simulink model "gm_uz_mpc_delay_comp"  (R2021a)
settings: Solver=FixedStepDiscrete  StartTime=0.0  StopTime=1/f  RelTol=1e-3
undefined symbols (not defined in the file or in its folder): A, f, Ld_over_LB, Lq_over_LB, omega_m, omegaB, psi_pm_over_psiB, Rs_over_ZB, t_ADC, Ts_times_ZB_over_Ld, Ts_times_ZB_over_Lq, Ts_times_ZB_over_Lx, Ts_times_ZB_over_Ly, v_dc, VB
libraries: hdlmdlgenlib x44, fl_lib x7, nesl_utility x7, simulink x4, ee_lib x2, hdlsllib x1
settings Model: Creator=micha  LastModifiedBy=micha
settings SolverCC: AlgebraicLoopSolver=TrustRegion
settings DataIOCC: LimitDataPoints=on  SaveOutput=off  SaveTime=off
settings OptimizationCC: BlockReduction=off  ConditionallyExecuteInputs=off  DefaultParameterBehavior=Inlined  LifeSpan=inf
settings DebuggingCC: AlgebraicLoopMsg=error  InheritedTsInSrcMsg=none  SingleTaskRateTransMsg=error  AllowSymbolicDim=off  StrictBusMsg=ErrorOnBusTreatedAsVector  SFUnexpectedBacktrackingDiag=warning  SFNoUnconditionalDefaultTransitionDiag=warning  SFExecutionAtInitializationDiag=none  SFMachineParentedDataDiag=warning  ArithmeticOperatorsInVariantConditions=warning
settings HardwareCC: ProdBitPerPointer=32  ProdBitPerSizeT=32  ProdBitPerPtrDiffT=32  ProdLargestAtomicFloat=None  ProdIntDivRoundTo=Undefined  ProdEndianess=Unspecified  ProdWordSize=32  ProdHWDeviceType=ASIC/FPGA->ASIC/FPGA  ProdEqTarget=off
settings SFSimCC: SimUseLocalCustomCode=off  CustomCodeUndefinedFunction=UseInterfaceOnly
settings RTWCC: RTWUseLocalCustomCode=off
settings CodeAppCC: StateflowObjectComments=on
settings GRTTargetCC: TargetLangStandard=C89/C90 (ANSI)
settings ConfigComp: CovScope=ReferencedModels  CovMetricSettings=dw  CovSaveCumulativeToWorkspaceVar=on  CovSaveSingleToWorkspaceVar=on  CovExternalEMLEnable=off  CovSFcnEnable=off

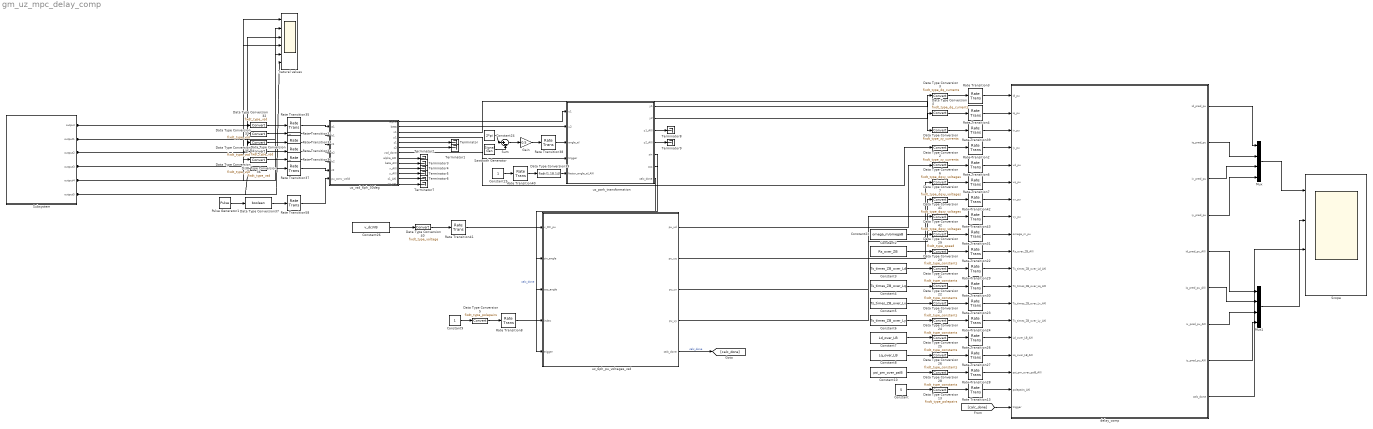
== system gm_uz_mpc_delay_comp ==
  Constant : Constant  Value=5
  Constant10 : Constant  Value=psi_pm_over_psiB
  Constant2 : Constant  Value=Rs_over_ZB
  Constant23 : Constant  Value=omega_m/omegaB
  Constant24 : Constant  Value=2*pi
  Constant25 : Constant
  Constant26 : Constant  Value=v_dc/VB
  Constant3 : Constant  Value=Ts_times_ZB_over_Ld
  Constant4 : Constant  Value=Ts_times_ZB_over_Lq
  Constant5 : Constant  Value=Ts_times_ZB_over_Lx
  Constant6 : Constant  Value=Ts_times_ZB_over_Ly
  Constant7 : Constant  Value=Ld_over_LB
  Constant8 : Constant  Value=Lq_over_LB
  Constant9 : Constant
  Data Type Conversion : DataTypeConversion  OutDataTypeStr=fixdt_type_xy_currents
  Data Type Conversion13 : DataTypeConversion  OutDataTypeStr=fixdt_type_polepairs
  Data Type Conversion2 : DataTypeConversion  OutDataTypeStr=fixdt_type_xy_currents
  Data Type Conversion{20..26,28} (8 alike) : DataTypeConversion  OutDataTypeStr=fixdt_type_constants
  Data Type Conversion29 : DataTypeConversion  OutDataTypeStr=fixdt_type_speed
  Data Type Conversion3 : DataTypeConversion  OutDataTypeStr=fixdt_type_dq_currents
  Data Type Conversion{32..36,38} (6 alike) : DataTypeConversion  OutDataTypeStr=fixdt_type_vsd
  Data Type Conversion37 : DataTypeConversion  OutDataTypeStr=boolean
  Data Type Conversion39 : DataTypeConversion  OutDataTypeStr=fixdt(1,18,14)
  Data Type Conversion4 : DataTypeConversion  OutDataTypeStr=fixdt_type_dq_currents
  Data Type Conversion40 : DataTypeConversion  OutDataTypeStr=fixdt_type_voltage
  Data Type Conversion{6..7,41..42} (4 alike) : DataTypeConversion  OutDataTypeStr=fixdt_type_dqxy_voltages
  Data Type Conversion5 : DataTypeConversion  OutDataTypeStr=fixdt_type_polepairs
  Gain : Gain  Gain=0.5
  Mux : Mux
  Mux1 : Mux
  Pulse Generator1 : DiscretePulseGenerator  PulseType=Time based  Period=t_ADC  PulseWidth=5
  Rate Transition{2..4,6..7,13,22..24,26..43,58} (28 alike) : RateTransition  OutPortSampleTime=t_clock
  Rate Transition8 : RateTransition  InitialCondition=1  OutPortSampleTime=t_clock
  Sawtooth Generator : SignalGenerator  WaveForm=sawtooth  Amplitude=2*pi  Frequency=2*pi*f  Units=rad/sec
  Scope : Scope  NumInputPorts=4
  Subsystem : Subsystem
  Sum : Sum  Inputs=|+-
  Terminator{,1..9} (10 alike) : Terminator
  delay_comp : Subsystem  TreatAsAtomicUnit=on
  natural values : Scope  NumInputPorts=6
  uz_6ph_pu_voltages_vsd : Subsystem
  uz_park_transformation : Subsystem  TreatAsAtomicUnit=on
  uz_vsd_6ph_30deg : Subsystem  TreatAsAtomicUnit=on
  wires:
  Data Type Conversion5/1 -> Rate Transition8/1
  Constant9/1 -> Data Type Conversion5/1
  Rate Transition8/1 -> uz_6ph_pu_voltages_vsd/4(index)
  delay_comp/9(calc_done) -> Scope/3
  Mux1/1 -> Scope/2
  delay_comp/5(id_pred_pu_AXI) -> Mux1/1
  delay_comp/7(ix_pred_pu_AXI) -> Mux1/3
  delay_comp/8(iy_pred_pu_AXI) -> Mux1/4
  delay_comp/6(iq_pred_pu_AXI) -> Mux1/2
  Mux/1 -> Scope/1
  delay_comp/4(iy_pred_pu) -> Mux/4
  delay_comp/3(ix_pred_pu) -> Mux/3
  delay_comp/2(iq_pred_pu) -> Mux/2
  delay_comp/1(id_pred_pu) -> Mux/1
  Rate Transition13/1 -> delay_comp/18(polepairs_AXI)
  Data Type Conversion13/1 -> Rate Transition13/1
  Constant/1 -> Data Type Conversion13/1
  Rate Transition28/1 -> delay_comp/17(psi_pm_over_psiB_AXI)
  Data Type Conversion28/1 -> Rate Transition28/1
  Constant10/1 -> Data Type Conversion28/1
  [calc_done] -> delay_comp/19(trigger)
  Rate Transition34/1 -> uz_vsd_6ph_30deg/4(a2)
  Data Type Conversion37/1 -> Rate Transition58/1
  Data Type Conversion36/1 -> Rate Transition36/1
  Constant26/1 -> Data Type Conversion40/1
  Data Type Conversion35/1 -> Rate Transition34/1
  uz_vsd_6ph_30deg/5(z1) -> Terminator/1
  uz_vsd_6ph_30deg/3(x1) -> Data Type Conversion/1
  Data Type Conversion32/1 -> Rate Transition35/1
  Data Type Conversion33/1 -> Rate Transition32/1
  Subsystem/6(output5) -> Data Type Conversion38/1, natural values/6
  Rate Transition32/1 -> uz_vsd_6ph_30deg/2(b1)
  Subsystem/3(output2) -> natural values/3, Data Type Conversion34/1
  Data Type Conversion34/1 -> Rate Transition33/1
  Rate Transition40/1 -> Data Type Conversion39/1
  Constant25/1 -> Rate Transition40/1
  Sawtooth Generator/1 -> Sum/2
  Rate Transition58/1 -> uz_vsd_6ph_30deg/7(pu_conv_valid)
  Sum/1 -> Gain/1
  Rate Transition36/1 -> uz_vsd_6ph_30deg/5(b2)
  Gain/1 -> Rate Transition38/1
  Subsystem/4(output3) -> natural values/4, Data Type Conversion35/1
  Data Type Conversion38/1 -> Rate Transition37/1
  Rate Transition38/1 -> uz_park_transformation/3(angle_el)
  uz_6ph_pu_voltages_vsd/1(pu_ud) -> Data Type Conversion6/1
  uz_6ph_pu_voltages_vsd/3(pu_ux) -> Data Type Conversion41/1
  Rate Transition33/1 -> uz_vsd_6ph_30deg/3(c1)
  uz_6ph_pu_voltages_vsd/5(calc_done) -> [calc_done]  "calc_done"
  Subsystem/5(output4) -> natural values/5, Data Type Conversion36/1
  uz_vsd_6ph_30deg/9(beta_AXI) -> Terminator3/1
  uz_park_transformation/1(y1) -> Data Type Conversion3/1
  uz_vsd_6ph_30deg/6(z2) -> Terminator1/1
  uz_vsd_6ph_30deg/10(x_AXI) -> Terminator4/1
  Rate Transition37/1 -> uz_vsd_6ph_30deg/6(c2)
  uz_vsd_6ph_30deg/4(y1) -> Data Type Conversion2/1
  Rate Transition41/1 -> uz_6ph_pu_voltages_vsd/1(v_DC_pu)
  uz_vsd_6ph_30deg/1(alpha) -> uz_park_transformation/1(u1)
  uz_park_transformation/6(cos) -> uz_6ph_pu_voltages_vsd/3(cos_angle)
  uz_park_transformation/7(calc_done) -> uz_6ph_pu_voltages_vsd/5(trigger)  "calc_done"
  Data Type Conversion39/1 -> uz_park_transformation/5(factor_angle_el_AXI)
  uz_6ph_pu_voltages_vsd/4(pu_uy) -> Data Type Conversion42/1
  uz_vsd_6ph_30deg/7(vsd_done) -> uz_park_transformation/4(trigger)
  Subsystem/2(output1) -> Data Type Conversion33/1, natural values/2
  Pulse Generator1/1 -> Data Type Conversion37/1
  uz_park_transformation/5(sin) -> uz_6ph_pu_voltages_vsd/2(sin_angle)
  Rate Transition35/1 -> uz_vsd_6ph_30deg/1(a1)
  uz_6ph_pu_voltages_vsd/2(pu_uq) -> Data Type Conversion7/1
  uz_vsd_6ph_30deg/2(beta) -> uz_park_transformation/2(u2)
  Constant24/1 -> Sum/1
  Data Type Conversion40/1 -> Rate Transition41/1
  Subsystem/1(output) -> Data Type Conversion32/1, natural values/1
  uz_park_transformation/2(y2) -> Data Type Conversion4/1
  uz_vsd_6ph_30deg/11(y_AXI) -> Terminator5/1
  uz_park_transformation/3(y1_AXI) -> Terminator8/1
  uz_vsd_6ph_30deg/13(z2_AXI) -> Terminator7/1
  uz_vsd_6ph_30deg/8(alpha_AXI) -> Terminator2/1
  uz_park_transformation/4(y2_AXI) -> Terminator9/1
  uz_vsd_6ph_30deg/12(z1_AXI) -> Terminator6/1
  Rate Transition43/1 -> delay_comp/8(vy_pu)
  Rate Transition7/1 -> delay_comp/6(vq_pu)
  Rate Transition6/1 -> delay_comp/5(vd_pu)
  Data Type Conversion42/1 -> Rate Transition43/1
  Data Type Conversion7/1 -> Rate Transition7/1
  Data Type Conversion41/1 -> Rate Transition42/1
  Rate Transition42/1 -> delay_comp/7(vx_pu)
  Data Type Conversion6/1 -> Rate Transition6/1
  Rate Transition39/1 -> delay_comp/3(ix_pu)
  Rate Transition4/1 -> delay_comp/2(iq_pu)
  Data Type Conversion2/1 -> Rate Transition2/1
  Data Type Conversion/1 -> Rate Transition39/1
  Data Type Conversion4/1 -> Rate Transition4/1
  Rate Transition3/1 -> delay_comp/1(id_pu)
  Data Type Conversion3/1 -> Rate Transition3/1
  Rate Transition2/1 -> delay_comp/4(iy_pu)
  Rate Transition31/1 -> delay_comp/9(omega_m_pu)
  Constant23/1 -> Data Type Conversion29/1
  Data Type Conversion29/1 -> Rate Transition31/1
  Constant7/1 -> Data Type Conversion25/1
  Constant4/1 -> Data Type Conversion22/1
  Constant5/1 -> Data Type Conversion23/1
  Rate Transition23/1 -> delay_comp/13(Ts_times_ZB_over_Lx_AXI)
  Data Type Conversion20/1 -> Rate Transition22/1
  Rate Transition24/1 -> delay_comp/14(Ts_times_ZB_over_Ly_AXI)
  Rate Transition26/1 -> delay_comp/15(Ld_over_LB_AXI)
  Data Type Conversion23/1 -> Rate Transition23/1
  Data Type Conversion22/1 -> Rate Transition30/1
  Data Type Conversion25/1 -> Rate Transition26/1
  Constant2/1 -> Data Type Conversion20/1
  Constant3/1 -> Data Type Conversion21/1
  Rate Transition27/1 -> delay_comp/16(Lq_over_LB_AXI)
  Rate Transition30/1 -> delay_comp/12(Ts_times_ZB_over_Lq_AXI)
  Constant6/1 -> Data Type Conversion24/1
  Data Type Conversion26/1 -> Rate Transition27/1
  Rate Transition29/1 -> delay_comp/11(Ts_times_ZB_over_Ld_AXI)
  Data Type Conversion21/1 -> Rate Transition29/1
  Rate Transition22/1 -> delay_comp/10(Rs_over_ZB_AXI)
  Constant8/1 -> Data Type Conversion26/1
  Data Type Conversion24/1 -> Rate Transition24/1

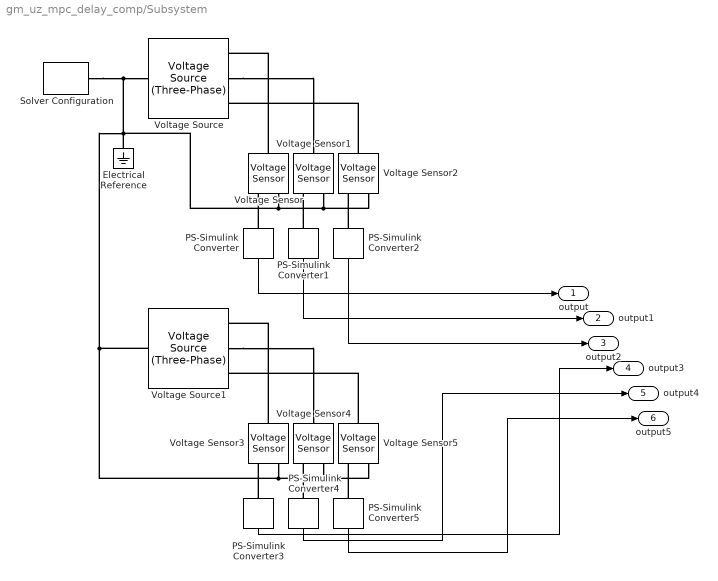
== system gm_uz_mpc_delay_comp/Subsystem ==
  Electrical Reference : fl_lib/Electrical/Electrical Elements/Electrical Reference
  PS-Simulink Converter{,1..5} (6 alike) : nesl_utility/PS-Simulink Converter  PhysicalDomain=network_engine_domain  SubClassName=ps_output  LeftPortType=input  RightPortType=output  PseudoPeriodic=off  Frequencies=[]  Unit=1  AffineConversion=off
  Solver Configuration : nesl_utility/Solver Configuration  PhysicalDomain=network_engine_domain  SubClassName=solver  LeftPortType=input  RightPortType=generic  Tones=[]  Harmonics=[]  SimulateNoise=off  Profile=off  UseLocalSampling=off  EnableSwitchedLinearOptims=on  FrequencyDomain=off  UseCCode=off  RelTol=0.001  AbsTol=1e-06  MinStep=1e-09  ToWorkspace=off  RevertToSquareIcSolve=off  NumHomotopyIterations=100  PhasorMode=off  PhasorModeNumHarmonics=1  DoDC=off  ResidualTolerance=1e-09  UseLocalSolver=on  LocalSolverChoice=NE_BACKWARD_EULER_ADVANCER  LocalSolverSampleTime=1e-6  DoFixedCost=on  MaxNonlinIter=3  MaxModeIter=2  ComputeImpulses=off  ImpulseIterations=2  LinearAlgebra=Sparse  EquationFormulation=NE_TIME_EF  DelaysMemoryBudget=1024  AutomaticFiltering=on  FilteringTimeConstant=0.001  PartitionStorageMethod=AS_NEEDED  PartitionMemoryBudget=1024  PartitionMethod=FAST
  Voltage Sensor{,1..5} (6 alike) : fl_lib/Electrical/Electrical Sensors/Voltage Sensor
  Voltage Source : ee_lib/Sources/Voltage Source (Three-Phase)  vline_rms=A*sqrt(3)/sqrt(2) V  shift=0 deg  freq=f Hz  impedance_option=1  SShortCircuit=1e6 V*A  XR=15  R=0.01 Ohm  L=3.97e-4 H  G_parasitic=0 1/Ohm  harmonic_option=1  harmonic_orders=Harmonic_Orders  harmonic_ratios=Harmonic_Amplitudes  I_specify=off  I_priority=None  I=[ 0 0 0 ] A  I_nominal_specify=off  I_nominal_unit=A  I_nominal_value=1
      settings: SourceProductBaseCode=PS  InternalSimscapePortConfiguration="{\"Bottom\":[],\"Left\":[{\"id\":\"n\",\"label\":\"n\",\"type\":\"foundation.electrical.electrical\"}],\"Right\":[{\"id\":\"a\",\"label\":\"a\",\"type\":\"foundation.electrical.electrical\"},{\"id\":\"b\",\"label\":\"b\",\"type\":\"foundation.electrical.electrical\"},{\"id\":\"c\",\"label\":\"c\",\"type\":\"foundation.electrical.electrical\"}],\"Top\":[]}"
  Voltage Source1 : ee_lib/Sources/Voltage Source (Three-Phase)  vline_rms=A*sqrt(3)/sqrt(2) V  shift=-30 deg  freq=f Hz  impedance_option=1  SShortCircuit=1e6 V*A  XR=15  R=0.01 Ohm  L=3.97e-4 H  G_parasitic=0 1/Ohm  harmonic_option=1  harmonic_orders=Harmonic_Orders  harmonic_ratios=Harmonic_Amplitudes  I_specify=off  I_priority=None  I=[ 0 0 0 ] A  I_nominal_specify=off  I_nominal_unit=A  I_nominal_value=1
      settings: SourceProductBaseCode=PS  InternalSimscapePortConfiguration="{\"Bottom\":[],\"Left\":[{\"id\":\"n\",\"label\":\"n\",\"type\":\"foundation.electrical.electrical\"}],\"Right\":[{\"id\":\"a\",\"label\":\"a\",\"type\":\"foundation.electrical.electrical\"},{\"id\":\"b\",\"label\":\"b\",\"type\":\"foundation.electrical.electrical\"},{\"id\":\"c\",\"label\":\"c\",\"type\":\"foundation.electrical.electrical\"}],\"Top\":[]}"
  output : Outport
  output1 : Outport  Port=2
  output2 : Outport  Port=3
  output3 : Outport  Port=4
  output4 : Outport  Port=5
  output5 : Outport  Port=6
  wires:
  PS-Simulink Converter2/1 -> output2/1
  PS-Simulink Converter5/1 -> output5/1
  PS-Simulink Converter1/1 -> output1/1
  PS-Simulink Converter4/1 -> output4/1
  PS-Simulink Converter3/1 -> output3/1
  PS-Simulink Converter/1 -> output/1
  connections:
  Voltage Source/RConn2 -- Voltage Sensor1/LConn1
  Voltage Sensor/LConn1 -- Voltage Source/RConn1
  PS-Simulink Converter3/LConn1 -- Voltage Sensor3/RConn1
  PS-Simulink Converter2/LConn1 -- Voltage Sensor2/RConn1
  Voltage Sensor2/LConn1 -- Voltage Source/RConn3
  PS-Simulink Converter4/LConn1 -- Voltage Sensor4/RConn1
  Voltage Sensor5/LConn1 -- Voltage Source1/RConn3
  Voltage Source1/RConn2 -- Voltage Sensor4/LConn1
  PS-Simulink Converter/LConn1 -- Voltage Sensor/RConn1
  Voltage Sensor3/LConn1 -- Voltage Source1/RConn1
  PS-Simulink Converter1/LConn1 -- Voltage Sensor1/RConn1
  PS-Simulink Converter5/LConn1 -- Voltage Sensor5/RConn1
  Voltage Sensor4/RConn2 -- Voltage Sensor3/RConn2 -- Voltage Source1/LConn1 -- Electrical Reference/LConn1 -- Voltage Sensor/RConn2 -- Voltage Sensor1/RConn2 -- Voltage Sensor2/RConn2 -- Voltage Source/LConn1 -- Solver Configuration/RConn1 -- Voltage Sensor5/RConn2

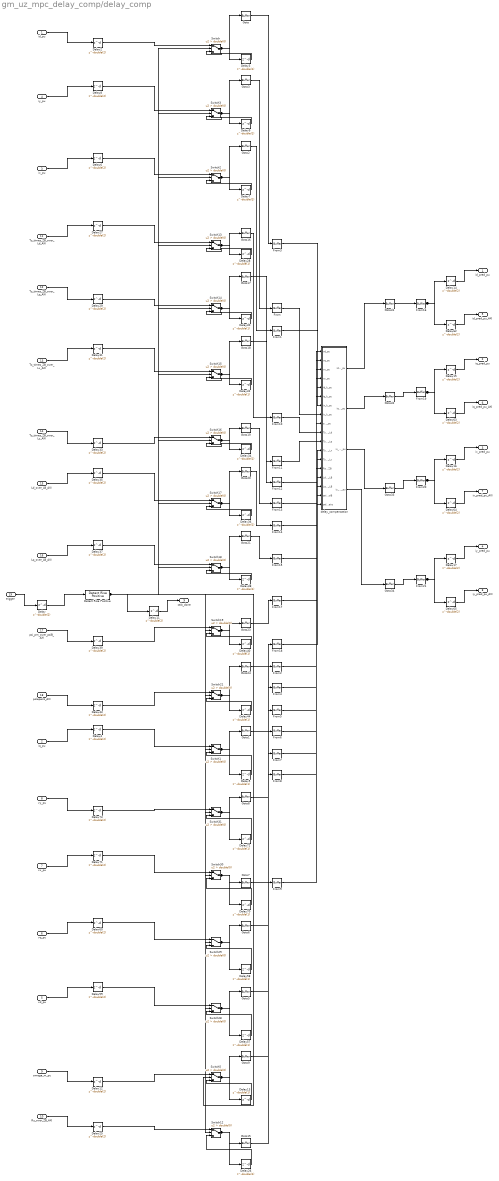
== system gm_uz_mpc_delay_comp/delay_comp ==
  id_pu : Inport  OutDataTypeStr=fixdt(1, 27, 16)  PortDimensions=1  SampleTime=1e-08
  iq_pu : Inport  Port=2  OutDataTypeStr=fixdt(1, 27, 16)  PortDimensions=1  SampleTime=1e-08
  ix_pu : Inport  Port=3  OutDataTypeStr=fixdt(1, 18, 11)  PortDimensions=1  SampleTime=1e-08
  iy_pu : Inport  Port=4  OutDataTypeStr=fixdt(1, 18, 11)  PortDimensions=1  SampleTime=1e-08
  vd_pu : Inport  Port=5  OutDataTypeStr=fixdt(1, 27, 24)  PortDimensions=1  SampleTime=1e-08
  vq_pu : Inport  Port=6  OutDataTypeStr=fixdt(1, 27, 24)  PortDimensions=1  SampleTime=1e-08
  vx_pu : Inport  Port=7  OutDataTypeStr=fixdt(1, 27, 24)  PortDimensions=1  SampleTime=1e-08
  vy_pu : Inport  Port=8  OutDataTypeStr=fixdt(1, 27, 24)  PortDimensions=1  SampleTime=1e-08
  omega_m_pu : Inport  Port=9  OutDataTypeStr=fixdt(1, 18, 15)  PortDimensions=1  SampleTime=1e-08
  Rs_over_ZB_AXI : Inport  Port=10  OutDataTypeStr=fixdt(1, 18, 15)  PortDimensions=1  SampleTime=1e-08
  Ts_times_ZB_over_Ld_AXI : Inport  Port=11  OutDataTypeStr=fixdt(1, 18, 15)  PortDimensions=1  SampleTime=1e-08
  Ts_times_ZB_over_Lq_AXI : Inport  Port=12  OutDataTypeStr=fixdt(1, 18, 15)  PortDimensions=1  SampleTime=1e-08
  Ts_times_ZB_over_Lx_AXI : Inport  Port=13  OutDataTypeStr=fixdt(1, 18, 15)  PortDimensions=1  SampleTime=1e-08
  Ts_times_ZB_over_Ly_AXI : Inport  Port=14  OutDataTypeStr=fixdt(1, 18, 15)  PortDimensions=1  SampleTime=1e-08
  Ld_over_LB_AXI : Inport  Port=15  OutDataTypeStr=fixdt(1, 18, 15)  PortDimensions=1  SampleTime=1e-08
  Lq_over_LB_AXI : Inport  Port=16  OutDataTypeStr=fixdt(1, 18, 15)  PortDimensions=1  SampleTime=1e-08
  psi_pm_over_psiB_AXI : Inport  Port=17  OutDataTypeStr=fixdt(1, 18, 15)  PortDimensions=1  SampleTime=1e-08
  polepairs_AXI : Inport  Port=18  OutDataTypeStr=uint32  PortDimensions=1  SampleTime=1e-08
  trigger : Inport  Port=19  OutDataTypeStr=boolean  PortDimensions=1  SampleTime=1e-08
  Delay{,2,4,6,8,11..12,14..17,25,27,29,31,33,35,37,39,43,59..60,62..65,71,73} (28 alike) : Delay  DelayLength=double(2)  InitialCondition=0  SampleTime=1e-08
  Delay{3,5,7,9,13,26,28,30,32,34,36,38,40,44,57..58,70,72} (18 alike) : Delay  DelayLength=double(1)  InitialCondition=0  SampleTime=1e-08
  Detect Rise Positive : simulink/Logic and Bit Operations/Detect Rise Positive  vinit=0  OutDataTypeStr=boolean
  From{,1..21} (22 alike) : hdlmdlgenlib/Buffer
      settings: SourceProductBaseCode=SL
  Goto{,1..3,5..9,15..21,23..24,31..34} (22 alike) : hdlmdlgenlib/Buffer
      settings: SourceProductBaseCode=SL
  Switch : Switch  Criteria=u2 > Threshold  Threshold=double(0)  OutDataTypeStr=fixdt(1, 27, 16)  SampleTime=1e-08
  Switch1 : Switch  Criteria=u2 > Threshold  Threshold=double(0)  OutDataTypeStr=fixdt(1, 27, 16)  SampleTime=1e-08
  Switch{5,12..19} (9 alike) : Switch  Criteria=u2 > Threshold  Threshold=double(0)  OutDataTypeStr=fixdt(1, 18, 15)  SampleTime=1e-08
  Switch2 : Switch  Criteria=u2 > Threshold  Threshold=double(0)  OutDataTypeStr=fixdt(1, 18, 11)  SampleTime=1e-08
  Switch21 : Switch  Criteria=u2 > Threshold  Threshold=double(0)  OutDataTypeStr=uint32  SampleTime=1e-08
  Switch{28..31} (4 alike) : Switch  Criteria=u2 > Threshold  Threshold=double(0)  OutDataTypeStr=fixdt(1, 27, 24)  SampleTime=1e-08
  Switch3 : Switch  Criteria=u2 > Threshold  Threshold=double(0)  OutDataTypeStr=fixdt(1, 18, 11)  SampleTime=1e-08
  delay_compensation : Subsystem
  id_pred_pu : Outport  SampleTime=1e-08
  iq_pred_pu : Outport  Port=2  SampleTime=1e-08
  ix_pred_pu : Outport  Port=3  SampleTime=1e-08
  iy_pred_pu : Outport  Port=4  SampleTime=1e-08
  id_pred_pu_AXI : Outport  Port=5  SampleTime=1e-08
  iq_pred_pu_AXI : Outport  Port=6  SampleTime=1e-08
  ix_pred_pu_AXI : Outport  Port=7  SampleTime=1e-08
  iy_pred_pu_AXI : Outport  Port=8  SampleTime=1e-08
  calc_done : Outport  Port=9  SampleTime=1e-08
  wires:
  id_pu/1 -> Delay2/1
  iq_pu/1 -> Delay4/1
  ix_pu/1 -> Delay6/1
  iy_pu/1 -> Delay8/1
  vd_pu/1 -> Delay59/1
  vq_pu/1 -> Delay60/1
  vx_pu/1 -> Delay71/1
  vy_pu/1 -> Delay73/1
  omega_m_pu/1 -> Delay12/1
  Rs_over_ZB_AXI/1 -> Delay25/1
  Ts_times_ZB_over_Ld_AXI/1 -> Delay27/1
  Ts_times_ZB_over_Lq_AXI/1 -> Delay29/1
  Ts_times_ZB_over_Lx_AXI/1 -> Delay31/1
  Ts_times_ZB_over_Ly_AXI/1 -> Delay33/1
  Ld_over_LB_AXI/1 -> Delay35/1
  Lq_over_LB_AXI/1 -> Delay37/1
  psi_pm_over_psiB_AXI/1 -> Delay39/1
  polepairs_AXI/1 -> Delay43/1
  trigger/1 -> Delay/1
  Delay/1 -> Detect Rise Positive/1
  Delay11/1 -> calc_done/1
  Delay12/1 -> Switch5/1
  Delay13/1 -> Switch5/3
  Delay14/1 -> id_pred_pu/1
  Delay15/1 -> iq_pred_pu/1
  Delay16/1 -> ix_pred_pu/1
  Delay17/1 -> iy_pred_pu/1
  Delay2/1 -> Switch/1
  Delay25/1 -> Switch12/1
  Delay26/1 -> Switch12/3
  Delay27/1 -> Switch13/1
  Delay28/1 -> Switch13/3
  Delay29/1 -> Switch14/1
  Delay3/1 -> Switch/3
  Delay30/1 -> Switch14/3
  Delay31/1 -> Switch15/1
  Delay32/1 -> Switch15/3
  Delay33/1 -> Switch16/1
  Delay34/1 -> Switch16/3
  Delay35/1 -> Switch17/1
  Delay36/1 -> Switch17/3
  Delay37/1 -> Switch18/1
  Delay38/1 -> Switch18/3
  Delay39/1 -> Switch19/1
  Delay4/1 -> Switch1/1
  Delay40/1 -> Switch19/3
  Delay43/1 -> Switch21/1
  Delay44/1 -> Switch21/3
  Delay5/1 -> Switch1/3
  Delay57/1 -> Switch28/3
  Delay58/1 -> Switch29/3
  Delay59/1 -> Switch28/1
  Delay6/1 -> Switch2/1
  Delay60/1 -> Switch29/1
  Delay62/1 -> id_pred_pu_AXI/1
  Delay63/1 -> iq_pred_pu_AXI/1
  Delay64/1 -> ix_pred_pu_AXI/1
  Delay65/1 -> iy_pred_pu_AXI/1
  Delay7/1 -> Switch2/3
  Delay70/1 -> Switch30/3
  Delay71/1 -> Switch30/1
  Delay72/1 -> Switch31/3
  Delay73/1 -> Switch31/1
  Delay8/1 -> Switch3/1
  Delay9/1 -> Switch3/3
  Detect Rise Positive/1 -> Switch5/2, Switch31/2, Switch30/2, Switch3/2, Switch29/2, Switch28/2, Switch21/2, Switch2/2, Switch19/2, Switch18/2, Switch17/2, Switch16/2, Switch15/2, Switch14/2, Switch13/2, Switch12/2, Switch1/2, Switch/2, Delay11/1
  From/1 -> delay_compensation/8(iy_k_pu)
  From1/1 -> delay_compensation/7(ix_k_pu)
  From10/1 -> delay_compensation/10(Ts_times_ZB_over_Ld)
  From11/1 -> delay_compensation/11(Ts_times_ZB_over_Lq)
  From12/1 -> delay_compensation/12(Ts_times_ZB_over_Lx)
  From13/1 -> delay_compensation/13(Ts_times_ZB_over_Ly)
  From14/1 -> delay_compensation/15(Ld_over_LB)
  From15/1 -> delay_compensation/16(Lq_over_LB)
  From16/1 -> Delay62/1, Delay14/1
  From17/1 -> delay_compensation/17(psi_pm_over_psiB)
  From18/1 -> delay_compensation/18(polepairs)
  From19/1 -> Delay63/1, Delay15/1
  From2/1 -> delay_compensation/6(iq_k_pu)
  From20/1 -> Delay64/1, Delay16/1
  From21/1 -> Delay65/1, Delay17/1
  From3/1 -> delay_compensation/5(id_k_pu)
  From4/1 -> delay_compensation/4(vy_pu)
  From5/1 -> delay_compensation/3(vx_pu)
  From6/1 -> delay_compensation/2(vq_pu)
  From7/1 -> delay_compensation/1(vd_pu)
  From8/1 -> delay_compensation/9(omega_m_pu)
  From9/1 -> delay_compensation/14(Rs_over_ZB)
  Switch/1 -> Goto/1, Delay3/1
  Switch1/1 -> Goto1/1, Delay5/1
  Switch12/1 -> Goto15/1, Delay26/1
  Switch13/1 -> Goto16/1, Delay28/1
  Switch14/1 -> Goto17/1, Delay30/1
  Switch15/1 -> Goto18/1, Delay32/1
  Switch16/1 -> Goto19/1, Delay34/1
  Switch17/1 -> Goto20/1, Delay36/1
  Switch18/1 -> Goto21/1, Delay38/1
  Switch19/1 -> Goto23/1, Delay40/1
  Switch2/1 -> Goto2/1, Delay7/1
  Switch21/1 -> Goto24/1, Delay44/1
  Switch28/1 -> Goto5/1, Delay57/1
  Switch29/1 -> Goto6/1, Delay58/1
  Switch3/1 -> Goto3/1, Delay9/1
  Switch30/1 -> Goto7/1, Delay70/1
  Switch31/1 -> Goto8/1, Delay72/1
  Switch5/1 -> Goto9/1, Delay13/1
  delay_compensation/1(id_delay_pu) -> Goto31/1
  delay_compensation/2(iq_delay_pu) -> Goto32/1
  delay_compensation/3(ix_delay_pu) -> Goto33/1
  delay_compensation/4(iy_delay_pu) -> Goto34/1
  Goto3/1 -> From/1
  Goto2/1 -> From1/1
  Goto16/1 -> From10/1
  Goto17/1 -> From11/1
  Goto18/1 -> From12/1
  Goto19/1 -> From13/1
  Goto20/1 -> From14/1
  Goto21/1 -> From15/1
  Goto31/1 -> From16/1
  Goto23/1 -> From17/1
  Goto24/1 -> From18/1
  Goto32/1 -> From19/1
  Goto1/1 -> From2/1
  Goto33/1 -> From20/1
  Goto34/1 -> From21/1
  Goto/1 -> From3/1
  Goto8/1 -> From4/1
  Goto7/1 -> From5/1
  Goto6/1 -> From6/1
  Goto5/1 -> From7/1
  Goto9/1 -> From8/1
  Goto15/1 -> From9/1

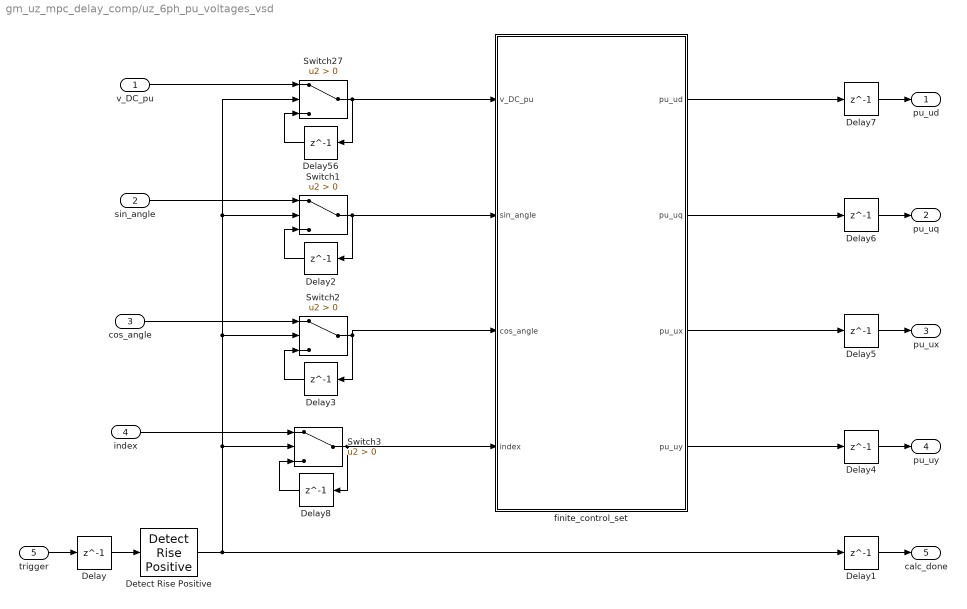
== system gm_uz_mpc_delay_comp/uz_6ph_pu_voltages_vsd ==
  v_DC_pu : Inport  OutDataTypeStr=fixdt_type_constants
  sin_angle : Inport  Port=2  OutDataTypeStr=fixdt_type_sin_cos
  cos_angle : Inport  Port=3  OutDataTypeStr=fixdt_type_sin_cos
  index : Inport  Port=4
  trigger : Inport  Port=5
  Delay{,1..7,56} (9 alike) : Delay  DelayLength=1
  Delay8 : Delay  DelayLength=1  InitialCondition=1
  Detect Rise Positive : simulink/Logic and Bit Operations/Detect Rise Positive  vinit=0  OutDataTypeStr=boolean
  Switch1 : Switch  Criteria=u2 > Threshold  OutDataTypeStr=fixdt_type_sin_cos
  Switch2 : Switch  Criteria=u2 > Threshold  OutDataTypeStr=fixdt_type_sin_cos
  Switch27 : Switch  Criteria=u2 > Threshold  OutDataTypeStr=fixdt_type_constants
  Switch3 : Switch  Criteria=u2 > Threshold  OutDataTypeStr=fixdt_type_polepairs
  finite_control_set : MATLAB Function  TreatAsAtomicUnit=on
  pu_ud : Outport
  pu_uq : Outport  Port=2
  pu_ux : Outport  Port=3
  pu_uy : Outport  Port=4
  calc_done : Outport  Port=5
  wires:
  Delay8/1 -> Switch3/3
  index/1 -> Switch3/1
  Switch3/1 -> Delay8/1, finite_control_set/4(index)
  Delay7/1 -> pu_ud/1
  Delay6/1 -> pu_uq/1
  Delay5/1 -> pu_ux/1
  Delay4/1 -> pu_uy/1
  Detect Rise Positive/1 -> Delay1/1, Switch27/2, Switch1/2, Switch2/2, Switch3/2
  Switch2/1 -> Delay3/1, finite_control_set/3(cos_angle)
  Delay3/1 -> Switch2/3
  cos_angle/1 -> Switch2/1
  Switch1/1 -> Delay2/1, finite_control_set/2(sin_angle)
  Delay2/1 -> Switch1/3
  sin_angle/1 -> Switch1/1
  Switch27/1 -> finite_control_set/1(v_DC_pu), Delay56/1
  v_DC_pu/1 -> Switch27/1
  Delay56/1 -> Switch27/3
  Delay1/1 -> calc_done/1
  Delay/1 -> Detect Rise Positive/1
  trigger/1 -> Delay/1
  finite_control_set/4(pu_uy) -> Delay4/1
  finite_control_set/3(pu_ux) -> Delay5/1
  finite_control_set/2(pu_uq) -> Delay6/1
  finite_control_set/1(pu_ud) -> Delay7/1

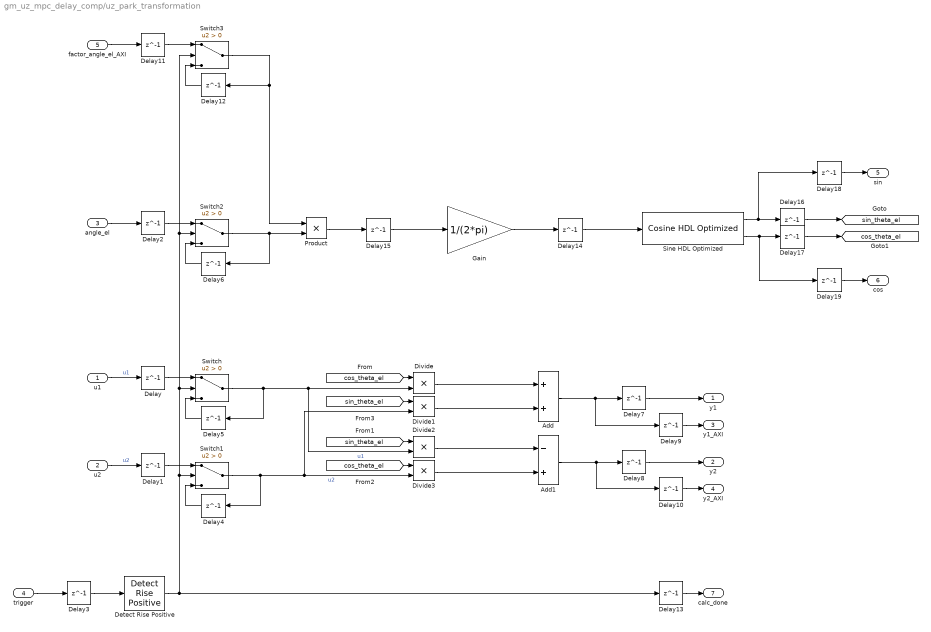
== system gm_uz_mpc_delay_comp/uz_park_transformation ==
  u1 : Inport
  u2 : Inport  Port=2
  angle_el : Inport  Port=3
  trigger : Inport  Port=4
  factor_angle_el_AXI : Inport  Port=5
  Add : Sum  OutDataTypeStr=fixdt(1,27,16)
  Add1 : Sum  Inputs=-+  OutDataTypeStr=fixdt(1,27,16)
  Delay{,1..19} (20 alike) : Delay  DelayLength=1
  Detect Rise Positive : simulink/Logic and Bit Operations/Detect Rise Positive  vinit=0  OutDataTypeStr=boolean
  Divide{,1..3} (4 alike) : Product  Inputs=**  OutDataTypeStr=fixdt(1,27,16)
  Gain : Gain  Gain=1/(2*pi)  OutDataTypeStr=fixdt(1,18,16)
  Product : Product  OutDataTypeStr=fixdt(1,18,14)
  Sine HDL Optimized : hdlsllib/Lookup Tables/Cosine HDL Optimized  OutputFormula=sin(2*pi*u) and cos(2*pi*u)  NumDataPoints=256  TableDataTypeStr=fixdt(0,17,16)  SimulateLUTROMDelay=off
      settings: SourceProductBaseCode=SL
  Switch{,1..3} (4 alike) : Switch  Criteria=u2 > Threshold
  y1 : Outport  VectorParamsAs1DForOutWhenUnconnected=off
  y2 : Outport  Port=2  VectorParamsAs1DForOutWhenUnconnected=off
  y1_AXI : Outport  Port=3  VectorParamsAs1DForOutWhenUnconnected=off
  y2_AXI : Outport  Port=4  VectorParamsAs1DForOutWhenUnconnected=off
  sin : Outport  Port=5  VectorParamsAs1DForOutWhenUnconnected=off
  cos : Outport  Port=6  VectorParamsAs1DForOutWhenUnconnected=off
  calc_done : Outport  Port=7  VectorParamsAs1DForOutWhenUnconnected=off
  tag scope: cos_theta_el=global, sin_theta_el=global
  wires:
  Delay19/1 -> cos/1
  Delay18/1 -> sin/1
  Delay17/1 -> [cos_theta_el]
  Delay16/1 -> [sin_theta_el]
  Delay14/1 -> Sine HDL Optimized/1
  Delay15/1 -> Gain/1
  Delay13/1 -> calc_done/1
  Delay3/1 -> Detect Rise Positive/1
  Product/1 -> Delay15/1
  Delay11/1 -> Switch3/1
  Delay12/1 -> Switch3/3
  Detect Rise Positive/1 -> Switch2/2, Switch3/2, Switch/2, Switch1/2, Delay13/1
  factor_angle_el_AXI/1 -> Delay11/1
  Switch3/1 -> Delay12/1, Product/1
  Switch2/1 -> Delay6/1, Product/2
  Delay10/1 -> y2_AXI/1
  Delay9/1 -> y1_AXI/1
  Delay8/1 -> y2/1
  Delay7/1 -> y1/1
  Delay6/1 -> Switch2/3
  Delay5/1 -> Switch/3
  Delay4/1 -> Switch1/3
  trigger/1 -> Delay3/1
  Delay2/1 -> Switch2/1
  Delay1/1 -> Switch1/1
  Delay/1 -> Switch/1
  u2/1 -> Delay1/1  "u2"
  u1/1 -> Delay/1  "u1"
  Gain/1 -> Delay14/1
  Sine HDL Optimized/1 -> Delay16/1, Delay18/1
  Sine HDL Optimized/2 -> Delay17/1, Delay19/1
  angle_el/1 -> Delay2/1
  Divide/1 -> Add/1
  Add1/1 -> Delay8/1, Delay10/1
  Add/1 -> Delay7/1, Delay9/1
  [sin_theta_el] -> Divide1/1
  [cos_theta_el] -> Divide/1
  Divide1/1 -> Add/2
  [sin_theta_el] -> Divide2/1
  Switch/1 -> Delay5/1, Divide/2, Divide2/2  "u1"
  [cos_theta_el] -> Divide3/1
  Divide3/1 -> Add1/2
  Divide2/1 -> Add1/1
  Switch1/1 -> Divide3/2, Divide1/2, Delay4/1  "u2"

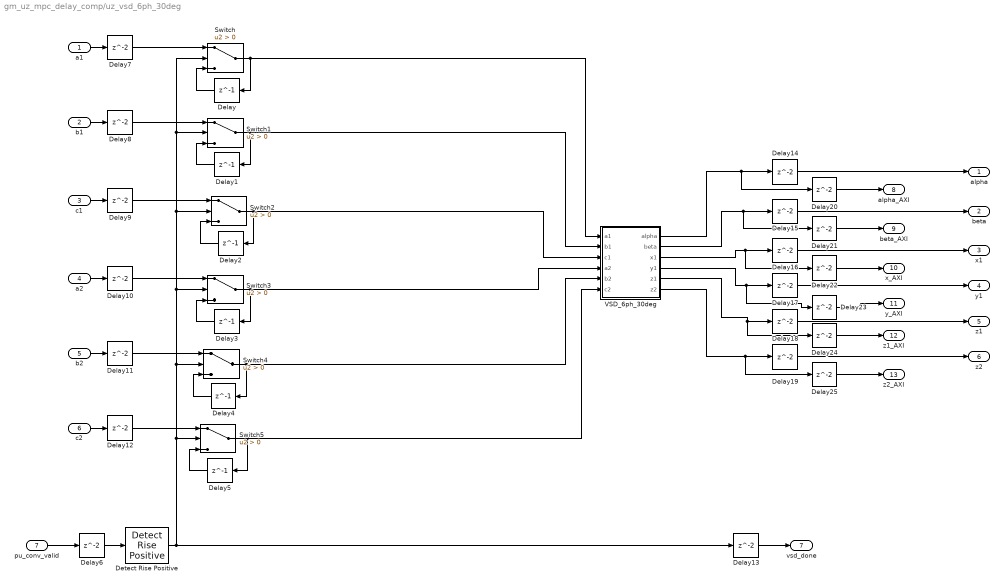
== system gm_uz_mpc_delay_comp/uz_vsd_6ph_30deg ==
  a1 : Inport
  b1 : Inport  Port=2
  c1 : Inport  Port=3
  a2 : Inport  Port=4
  b2 : Inport  Port=5
  c2 : Inport  Port=6
  pu_conv_valid : Inport  Port=7
  Delay{,1..5} (6 alike) : Delay  DelayLength=1
  Delay{6..25} (20 alike) : Delay
  Detect Rise Positive : simulink/Logic and Bit Operations/Detect Rise Positive  vinit=0  OutDataTypeStr=boolean
  Switch{,1..5} (6 alike) : Switch  Criteria=u2 > Threshold  OutDataTypeStr=fixdt_type_vsd
  VSD_6ph_30deg : MATLAB Function  TreatAsAtomicUnit=on
  alpha : Outport  OutDataTypeStr=fixdt(1,18,11)  VectorParamsAs1DForOutWhenUnconnected=off
  beta : Outport  Port=2  OutDataTypeStr=fixdt(1,18,11)  VectorParamsAs1DForOutWhenUnconnected=off
  x1 : Outport  Port=3  OutDataTypeStr=fixdt(1,18,11)  VectorParamsAs1DForOutWhenUnconnected=off
  y1 : Outport  Port=4  OutDataTypeStr=fixdt(1,18,11)  VectorParamsAs1DForOutWhenUnconnected=off
  z1 : Outport  Port=5  OutDataTypeStr=fixdt(1,18,11)  VectorParamsAs1DForOutWhenUnconnected=off
  z2 : Outport  Port=6  OutDataTypeStr=fixdt(1,18,11)  VectorParamsAs1DForOutWhenUnconnected=off
  vsd_done : Outport  Port=7  VectorParamsAs1DForOutWhenUnconnected=off
  alpha_AXI : Outport  Port=8  OutDataTypeStr=fixdt(1,18,11)  VectorParamsAs1DForOutWhenUnconnected=off
  beta_AXI : Outport  Port=9  OutDataTypeStr=fixdt(1,18,11)  VectorParamsAs1DForOutWhenUnconnected=off
  x_AXI : Outport  Port=10  OutDataTypeStr=fixdt(1,18,11)  VectorParamsAs1DForOutWhenUnconnected=off
  y_AXI : Outport  Port=11  OutDataTypeStr=fixdt(1,18,11)  VectorParamsAs1DForOutWhenUnconnected=off
  z1_AXI : Outport  Port=12  OutDataTypeStr=fixdt(1,18,11)  VectorParamsAs1DForOutWhenUnconnected=off
  z2_AXI : Outport  Port=13  OutDataTypeStr=fixdt(1,18,11)  VectorParamsAs1DForOutWhenUnconnected=off
  wires:
  Delay25/1 -> z2_AXI/1
  Delay24/1 -> z1_AXI/1
  Delay23/1 -> y_AXI/1
  Delay22/1 -> x_AXI/1
  Delay21/1 -> beta_AXI/1
  Delay20/1 -> alpha_AXI/1
  Delay19/1 -> z2/1
  Delay18/1 -> z1/1
  Delay17/1 -> y1/1
  Delay16/1 -> x1/1
  Delay15/1 -> beta/1
  Delay14/1 -> alpha/1
  Delay13/1 -> vsd_done/1
  Delay12/1 -> Switch5/1
  Delay11/1 -> Switch4/1
  Delay10/1 -> Switch3/1
  Delay9/1 -> Switch2/1
  Delay8/1 -> Switch1/1
  Delay7/1 -> Switch/1
  Delay6/1 -> Detect Rise Positive/1
  c2/1 -> Delay12/1
  b2/1 -> Delay11/1
  a2/1 -> Delay10/1
  c1/1 -> Delay9/1
  b1/1 -> Delay8/1
  a1/1 -> Delay7/1
  Switch5/1 -> Delay5/1, VSD_6ph_30deg/6(c2)
  Delay5/1 -> Switch5/3
  Switch4/1 -> Delay4/1, VSD_6ph_30deg/5(b2)
  Delay4/1 -> Switch4/3
  Switch3/1 -> Delay3/1, VSD_6ph_30deg/4(a2)
  Delay3/1 -> Switch3/3
  Switch2/1 -> Delay2/1, VSD_6ph_30deg/3(c1)
  Delay2/1 -> Switch2/3
  Switch1/1 -> Delay1/1, VSD_6ph_30deg/2(b1)
  Delay1/1 -> Switch1/3
  Switch/1 -> Delay/1, VSD_6ph_30deg/1(a1)
  Delay/1 -> Switch/3
  Detect Rise Positive/1 -> Delay13/1, Switch/2, Switch1/2, Switch2/2, Switch3/2, Switch4/2, Switch5/2
  pu_conv_valid/1 -> Delay6/1
  VSD_6ph_30deg/6(z2) -> Delay19/1, Delay25/1
  VSD_6ph_30deg/5(z1) -> Delay18/1, Delay24/1
  VSD_6ph_30deg/4(y1) -> Delay17/1, Delay23/1
  VSD_6ph_30deg/3(x1) -> Delay16/1, Delay22/1
  VSD_6ph_30deg/2(beta) -> Delay15/1, Delay21/1
  VSD_6ph_30deg/1(alpha) -> Delay14/1, Delay20/1

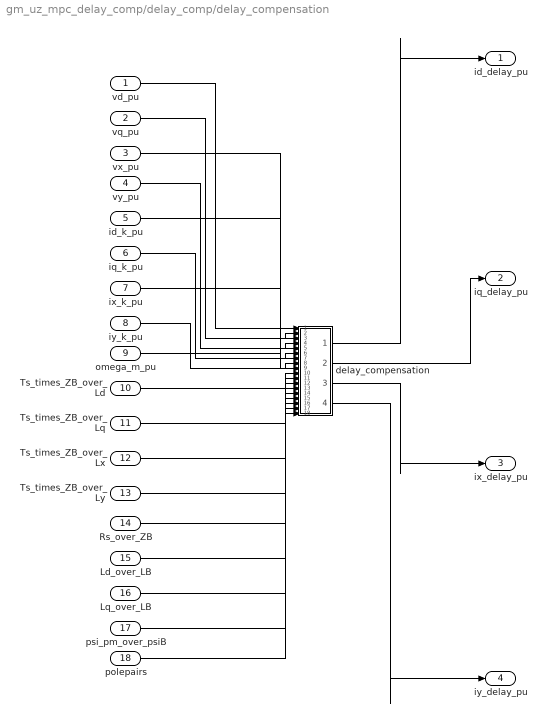
== system gm_uz_mpc_delay_comp/delay_comp/delay_compensation ==
  vd_pu : Inport  OutDataTypeStr=fixdt(1, 27, 24)  PortDimensions=1  SampleTime=1e-08
  vq_pu : Inport  Port=2  OutDataTypeStr=fixdt(1, 27, 24)  PortDimensions=1  SampleTime=1e-08
  vx_pu : Inport  Port=3  OutDataTypeStr=fixdt(1, 27, 24)  PortDimensions=1  SampleTime=1e-08
  vy_pu : Inport  Port=4  OutDataTypeStr=fixdt(1, 27, 24)  PortDimensions=1  SampleTime=1e-08
  id_k_pu : Inport  Port=5  OutDataTypeStr=fixdt(1, 27, 16)  PortDimensions=1  SampleTime=1e-08
  iq_k_pu : Inport  Port=6  OutDataTypeStr=fixdt(1, 27, 16)  PortDimensions=1  SampleTime=1e-08
  ix_k_pu : Inport  Port=7  OutDataTypeStr=fixdt(1, 18, 11)  PortDimensions=1  SampleTime=1e-08
  iy_k_pu : Inport  Port=8  OutDataTypeStr=fixdt(1, 18, 11)  PortDimensions=1  SampleTime=1e-08
  omega_m_pu : Inport  Port=9  OutDataTypeStr=fixdt(1, 18, 15)  PortDimensions=1  SampleTime=1e-08
  Ts_times_ZB_over_Ld : Inport  Port=10  OutDataTypeStr=fixdt(1, 18, 15)  PortDimensions=1  SampleTime=1e-08
  Ts_times_ZB_over_Lq : Inport  Port=11  OutDataTypeStr=fixdt(1, 18, 15)  PortDimensions=1  SampleTime=1e-08
  Ts_times_ZB_over_Lx : Inport  Port=12  OutDataTypeStr=fixdt(1, 18, 15)  PortDimensions=1  SampleTime=1e-08
  Ts_times_ZB_over_Ly : Inport  Port=13  OutDataTypeStr=fixdt(1, 18, 15)  PortDimensions=1  SampleTime=1e-08
  Rs_over_ZB : Inport  Port=14  OutDataTypeStr=fixdt(1, 18, 15)  PortDimensions=1  SampleTime=1e-08
  Ld_over_LB : Inport  Port=15  OutDataTypeStr=fixdt(1, 18, 15)  PortDimensions=1  SampleTime=1e-08
  Lq_over_LB : Inport  Port=16  OutDataTypeStr=fixdt(1, 18, 15)  PortDimensions=1  SampleTime=1e-08
  psi_pm_over_psiB : Inport  Port=17  OutDataTypeStr=fixdt(1, 18, 15)  PortDimensions=1  SampleTime=1e-08
  polepairs : Inport  Port=18  OutDataTypeStr=uint32  PortDimensions=1  SampleTime=1e-08
  delay_compensation : MATLAB Function  TreatAsAtomicUnit=on
  id_delay_pu : Outport  SampleTime=1e-08  VectorParamsAs1DForOutWhenUnconnected=off
  iq_delay_pu : Outport  Port=2  SampleTime=1e-08
  ix_delay_pu : Outport  Port=3  SampleTime=1e-08
  iy_delay_pu : Outport  Port=4  SampleTime=1e-08
  wires:
  vd_pu/1 -> delay_compensation/1(vd_pu)
  vq_pu/1 -> delay_compensation/2(vq_pu)
  vx_pu/1 -> delay_compensation/3(vx_pu)
  vy_pu/1 -> delay_compensation/4(vy_pu)
  id_k_pu/1 -> delay_compensation/5(id_k_pu)
  iq_k_pu/1 -> delay_compensation/6(iq_k_pu)
  ix_k_pu/1 -> delay_compensation/7(ix_k_pu)
  iy_k_pu/1 -> delay_compensation/8(iy_k_pu)
  omega_m_pu/1 -> delay_compensation/9(omega_m_pu)
  Ts_times_ZB_over_Ld/1 -> delay_compensation/10(Ts_times_ZB_over_Ld)
  Ts_times_ZB_over_Lq/1 -> delay_compensation/11(Ts_times_ZB_over_Lq)
  Ts_times_ZB_over_Lx/1 -> delay_compensation/12(Ts_times_ZB_over_Lx)
  Ts_times_ZB_over_Ly/1 -> delay_compensation/13(Ts_times_ZB_over_Ly)
  Rs_over_ZB/1 -> delay_compensation/14(Rs_over_ZB)
  Ld_over_LB/1 -> delay_compensation/15(Ld_over_LB)
  Lq_over_LB/1 -> delay_compensation/16(Lq_over_LB)
  psi_pm_over_psiB/1 -> delay_compensation/17(psi_pm_over_psiB)
  polepairs/1 -> delay_compensation/18(polepairs)
  delay_compensation/1(id_delay_pu) -> id_delay_pu/1
  delay_compensation/2(iq_delay_pu) -> iq_delay_pu/1
  delay_compensation/3(ix_delay_pu) -> ix_delay_pu/1
  delay_compensation/4(iy_delay_pu) -> iy_delay_pu/1

== matlab function gm_uz_mpc_delay_comp/delay_comp/delay_compensation/delay_compensation ==
  settings: fimath=fimath('RoundingMethod', 'Floor','OverflowAction', 'Wrap','ProductMode', 'FullPrecision', 'SumMode', 'FullPrecision')
  data: vd_pu input; id_delay_pu output; vq_pu input; vx_pu input; vy_pu input; id_k_pu input; iq_k_pu input; ix_k_pu input; iy_k_pu input; omega_m_pu input; Ts_times_ZB_over_Ld input; Ts_times_ZB_over_Lq input; Ts_times_ZB_over_Lx input; Ts_times_ZB_over_Ly input; Rs_over_ZB input; Ld_over_LB input; Lq_over_LB input; psi_pm_over_psiB input; polepairs input; iq_delay_pu output; ix_delay_pu output; iy_delay_pu output
function [id_delay_pu,iq_delay_pu,ix_delay_pu,iy_delay_pu] = predict_currents(vd_pu,vq_pu,vx_pu,vy_pu,id_k_pu,iq_k_pu,ix_k_pu,iy_k_pu,...
                                                                                        omega_m_pu,Ts_times_ZB_over_Ld,Ts_times_ZB_over_Lq,...
                                                                                        Ts_times_ZB_over_Lx,Ts_times_ZB_over_Ly,Rs_over_ZB,Ld_over_LB,...
                                                                                        Lq_over_LB,psi_pm_over_psiB,polepairs)                                                                     
    
    fm = fimath();
    vd_pu = fi(vd_pu,1,27,24,fm);
    vq_pu = fi(vq_pu,1,27,24,fm);
    vx_pu = fi(vx_pu,1,27,24,fm);
    vy_pu = fi(vy_pu,1,27,24,fm);
    
    id_k_pu = fi(id_k_pu,1,27,16,fm);
    iq_k_pu = fi(iq_k_pu,1,27,16,fm);
    ix_k_pu = fi(ix_k_pu,1,27,16,fm);
    iy_k_pu = fi(iy_k_pu,1,27,16,fm);
    
    omega_m_pu = fi(omega_m_pu,1,18,15,fm);
    
    Ts_times_ZB_over_Ld = fi(Ts_times_ZB_over_Ld,1,18,15,fm);
    Ts_times_ZB_over_Lq = fi(Ts_times_ZB_over_Lq,1,18,15,fm);
    Ts_times_ZB_over_Lx = fi(Ts_times_ZB_over_Lx,1,18,15,fm);
    Ts_times_ZB_over_Ly = fi(Ts_times_ZB_over_Ly,1,18,15,fm);
    Rs_over_ZB = fi(Rs_over_ZB,1,18,15,fm);
    Ld_over_LB = fi(Ld_over_LB,1,18,15,fm);
    Lq_over_LB = fi(Lq_over_LB,1,18,15,fm);
    psi_pm_over_psiB = fi(psi_pm_over_psiB,1,18,15,fm);
    polepairs = fi(polepairs,0,18,0,fm);
        
    %Prediction d-current
    id_delay_pu = fi(Ts_times_ZB_over_Ld *(vd_pu - Rs_over_ZB * id_k_pu + iq_k_pu * Lq_over_LB * omega_m_pu * polepairs) + id_k_pu,1,27,24);
    
    %Prediction q-current
    iq_delay_pu = fi(Ts_times_ZB_over_Lq *(vq_pu - Rs_over_ZB * iq_k_pu - omega_m_pu * polepairs * Ld_over_LB * id_k_pu - omega_m_pu * polepairs * psi_pm_over_psiB) + iq_k_pu,1,27,24);
       
    %Prediction x-current
    ix_delay_pu = fi(Ts_times_ZB_over_Lx *(vx_pu - Rs_over_ZB* ix_k_pu) + ix_k_pu,1,27,24);
   
    %Prediction y-current
    iy_delay_pu = fi(Ts_times_ZB_over_Ly *(vy_pu - Rs_over_ZB * iy_k_pu) + iy_k_pu,1,27,24);
  
end

== matlab function gm_uz_mpc_delay_comp/uz_vsd_6ph_30deg/VSD_6ph_30deg ==
  settings: fimath=fimath('RoundingMethod', 'Floor','OverflowAction', 'Wrap','ProductMode', 'FullPrecision', 'SumMode', 'FullPrecision')
  data: a1 input; alpha output; b1 input; c1 input; a2 input; b2 input; c2 input; beta output; x1 output; y1 output; z1 output; z2 output
function [alpha,beta,x1,y1,z1,z2] = fcn(a1,b1,c1,a2,b2,c2)


A = [fi(0,1,18,11) fi(0,1,18,11) fi(0,1,18,11) fi(0,1,18,11) fi(0,1,18,11) fi(0,1,18,11)]';

A =    2/6*[1    -0.5        -0.5        sqrt(3)/2   -sqrt(3)/2  0 ;
           0    sqrt(3)/2   -sqrt(3)/2  0.5         0.5         -1;
           1    -0.5        -0.5        -sqrt(3)/2  sqrt(3)/2   0 ;
           0    -sqrt(3)/2  sqrt(3)/2   0.5         0.5         -1;
           0.5   0.5          0.5          0           0           0 ;
           0    0           0           0.5          0.5          0.5] * [a1 b1 c1 a2 b2 c2]';

alpha = fi(A(1),1,18,11);
beta = fi(A(2),1,18,11);
x1 = fi(A(3),1,18,11);
y1 = fi(A(4),1,18,11);
z1 = fi(A(5),1,18,11);
z2 = fi(A(6),1,18,11);

== matlab function gm_uz_mpc_delay_comp/uz_6ph_pu_voltages_vsd/finite_control_set ==
  data: v_DC_pu input; sin_angle input; pu_ud output; pu_uq output; pu_ux output; pu_uy output; cos_angle input; index input
function [pu_ud,pu_uq,pu_ux,pu_uy] = voltage_space_vectors(v_DC_pu, sin_angle, cos_angle, index)

fm = fimath();
v_DC_pu = fi(v_DC_pu,1,18,15,fm);

% u_d-voltages
vd_pu = v_DC_pu * fi([0.000000*cos_angle + 0.000000*sin_angle;
0.333333*cos_angle + -0.000000*sin_angle;
-0.166667*cos_angle + 0.288675*sin_angle;
0.166667*cos_angle + 0.288675*sin_angle;
-0.166667*cos_angle + -0.288675*sin_angle;
0.166667*cos_angle + -0.288675*sin_angle;
-0.333333*cos_angle + 0.000000*sin_angle;
0.000000*cos_angle + 0.000000*sin_angle;
0.288675*cos_angle + 0.166667*sin_angle;
0.622008*cos_angle + 0.166667*sin_angle;
0.122008*cos_angle + 0.455342*sin_angle;
0.455342*cos_angle + 0.455342*sin_angle;
0.122008*cos_angle + -0.122008*sin_angle;
0.455342*cos_angle + -0.122008*sin_angle;
-0.044658*cos_angle + 0.166667*sin_angle;
0.288675*cos_angle + 0.166667*sin_angle;
-0.288675*cos_angle + 0.166667*sin_angle;
0.044658*cos_angle + 0.166667*sin_angle;
-0.455342*cos_angle + 0.455342*sin_angle;
-0.122008*cos_angle + 0.455342*sin_angle;
-0.455342*cos_angle + -0.122008*sin_angle;
-0.122008*cos_angle + -0.122008*sin_angle;
-0.622008*cos_angle + 0.166667*sin_angle;
-0.288675*cos_angle + 0.166667*sin_angle;
0.000000*cos_angle + 0.333333*sin_angle;
0.333333*cos_angle + 0.333333*sin_angle;
-0.166667*cos_angle + 0.622008*sin_angle;
0.166667*cos_angle + 0.622008*sin_angle;
-0.166667*cos_angle + 0.044658*sin_angle;
0.166667*cos_angle + 0.044658*sin_angle;
-0.333333*cos_angle + 0.333333*sin_angle;
0.000000*cos_angle + 0.333333*sin_angle;
-0.000000*cos_angle + -0.333333*sin_angle;
0.333333*cos_angle + -0.333333*sin_angle;
-0.166667*cos_angle + -0.044658*sin_angle;
0.166667*cos_angle + -0.044658*sin_angle;
-0.166667*cos_angle + -0.622008*sin_angle;
0.166667*cos_angle + -0.622008*sin_angle;
-0.333333*cos_angle + -0.333333*sin_angle;
-0.000000*cos_angle + -0.333333*sin_angle;
0.288675*cos_angle + -0.166667*sin_angle;
0.622008*cos_angle + -0.166667*sin_angle;
0.122008*cos_angle + 0.122008*sin_angle;
0.455342*cos_angle + 0.122008*sin_angle;
0.122008*cos_angle + -0.455342*sin_angle;
0.455342*cos_angle + -0.455342*sin_angle;
-0.044658*cos_angle + -0.166667*sin_angle;
0.288675*cos_angle + -0.166667*sin_angle;
-0.288675*cos_angle + -0.166667*sin_angle;
0.044658*cos_angle + -0.166667*sin_angle;
-0.455342*cos_angle + 0.122008*sin_angle;
-0.122008*cos_angle + 0.122008*sin_angle;
-0.455342*cos_angle + -0.455342*sin_angle;
-0.122008*cos_angle + -0.455342*sin_angle;
-0.622008*cos_angle + -0.166667*sin_angle;
-0.288675*cos_angle + -0.166667*sin_angle;
0.000000*cos_angle + 0.000000*sin_angle;
0.333333*cos_angle + -0.000000*sin_angle;
-0.166667*cos_angle + 0.288675*sin_angle;
0.166667*cos_angle + 0.288675*sin_angle;
-0.166667*cos_angle + -0.288675*sin_angle;
0.166667*cos_angle + -0.288675*sin_angle;
-0.333333*cos_angle + 0.000000*sin_angle;
0.000000*cos_angle + 0.000000*sin_angle],1,18,15);

% u_q-voltages
vq_pu = v_DC_pu * fi([0.000000*-sin_angle + 0.000000*cos_angle;
0.333333*-sin_angle + -0.000000*cos_angle;
-0.166667*-sin_angle + 0.288675*cos_angle;
0.166667*-sin_angle + 0.288675*cos_angle;
-0.166667*-sin_angle + -0.288675*cos_angle;
0.166667*-sin_angle + -0.288675*cos_angle;
-0.333333*-sin_angle + 0.000000*cos_angle;
0.000000*-sin_angle + 0.000000*cos_angle;
0.288675*-sin_angle + 0.166667*cos_angle;
0.622008*-sin_angle + 0.166667*cos_angle;
0.122008*-sin_angle + 0.455342*cos_angle;
0.455342*-sin_angle + 0.455342*cos_angle;
0.122008*-sin_angle + -0.122008*cos_angle;
0.455342*-sin_angle + -0.122008*cos_angle;
-0.044658*-sin_angle + 0.166667*cos_angle;
0.288675*-sin_angle + 0.166667*cos_angle;
-0.288675*-sin_angle + 0.166667*cos_angle;
0.044658*-sin_angle + 0.166667*cos_angle;
-0.455342*-sin_angle + 0.455342*cos_angle;
-0.122008*-sin_angle + 0.455342*cos_angle;
-0.455342*-sin_angle + -0.122008*cos_angle;
-0.122008*-sin_angle + -0.122008*cos_angle;
-0.622008*-sin_angle + 0.166667*cos_angle;
-0.288675*-sin_angle + 0.166667*cos_angle;
0.000000*-sin_angle + 0.333333*cos_angle;
0.333333*-sin_angle + 0.333333*cos_angle;
-0.166667*-sin_angle + 0.622008*cos_angle;
0.166667*-sin_angle + 0.622008*cos_angle;
-0.166667*-sin_angle + 0.044658*cos_angle;
0.166667*-sin_angle + 0.044658*cos_angle;
-0.333333*-sin_angle + 0.333333*cos_angle;
0.000000*-sin_angle + 0.333333*cos_angle;
-0.000000*-sin_angle + -0.333333*cos_angle;
0.333333*-sin_angle + -0.333333*cos_angle;
-0.166667*-sin_angle + -0.044658*cos_angle;
0.166667*-sin_angle + -0.044658*cos_angle;
-0.166667*-sin_angle + -0.622008*cos_angle;
0.166667*-sin_angle + -0.622008*cos_angle;
-0.333333*-sin_angle + -0.333333*cos_angle;
-0.000000*-sin_angle + -0.333333*cos_angle;
0.288675*-sin_angle + -0.166667*cos_angle;
0.622008*-sin_angle + -0.166667*cos_angle;
0.122008*-sin_angle + 0.122008*cos_angle;
0.455342*-sin_angle + 0.122008*cos_angle;
0.122008*-sin_angle + -0.455342*cos_angle;
0.455342*-sin_angle + -0.455342*cos_angle;
-0.044658*-sin_angle + -0.166667*cos_angle;
0.288675*-sin_angle + -0.166667*cos_angle;
-0.288675*-sin_angle + -0.166667*cos_angle;
0.044658*-sin_angle + -0.166667*cos_angle;
-0.455342*-sin_angle + 0.122008*cos_angle;
-0.122008*-sin_angle + 0.122008*cos_angle;
-0.455342*-sin_angle + -0.455342*cos_angle;
-0.122008*-sin_angle + -0.455342*cos_angle;
-0.622008*-sin_angle + -0.166667*cos_angle;
-0.288675*-sin_angle + -0.166667*cos_angle;
0.000000*-sin_angle + 0.000000*cos_angle;
0.333333*-sin_angle + -0.000000*cos_angle;
-0.166667*-sin_angle + 0.288675*cos_angle;
0.166667*-sin_angle + 0.288675*cos_angle;
-0.166667*-sin_angle + -0.288675*cos_angle;
0.166667*-sin_angle + -0.288675*cos_angle;
-0.333333*-sin_angle + 0.000000*cos_angle;
0.000000*-sin_angle + 0.000000*cos_angle],1,18,15);
     
% u_x-voltages
vx_pu = v_DC_pu * fi([0.000000;
0.333333;
-0.166667;
0.166667;
-0.166667;
0.166667;
-0.333333;
0.000000;
-0.288675;
0.044658;
-0.455342;
-0.122008;
-0.455342;
-0.122008;
-0.622008;
-0.288675;
0.288675;
0.622008;
0.122008;
0.455342;
0.122008;
0.455342;
-0.044658;
0.288675;
0.000000;
0.333333;
-0.166667;
0.166667;
-0.166667;
0.166667;
-0.333333;
0.000000;
-0.000000;
0.333333;
-0.166667;
0.166667;
-0.166667;
0.166667;
-0.333333;
-0.000000;
-0.288675;
0.044658;
-0.455342;
-0.122008;
-0.455342;
-0.122008;
-0.622008;
-0.288675;
0.288675;
0.622008;
0.122008;
0.455342;
0.122008;
0.455342;
-0.044658;
0.288675;
0.000000;
0.333333;
-0.166667;
0.166667;
-0.166667;
0.166667;
-0.333333;
0.000000],1,18,15);

% u_y-voltages
vy_pu = v_DC_pu * fi([0.000000;
-0.000000;
-0.288675;
-0.288675;
0.288675;
0.288675;
0.000000;
0.000000;
0.166667;
0.166667;
-0.122008;
-0.122008;
0.455342;
0.455342;
0.166667;
0.166667;
0.166667;
0.166667;
-0.122008;
-0.122008;
0.455342;
0.455342;
0.166667;
0.166667;
0.333333;
0.333333;
0.044658;
0.044658;
0.622008;
0.622008;
0.333333;
0.333333;
-0.333333;
-0.333333;
-0.622008;
-0.622008;
-0.044658;
-0.044658;
-0.333333;
-0.333333;
-0.166667;
-0.166667;
-0.455342;
-0.455342;
0.122008;
0.122008;
-0.166667;
-0.166667;
-0.166667;
-0.166667;
-0.455342;
-0.455342;
0.122008;
0.122008;
-0.166667;
-0.166667;
0.000000;
-0.000000;
-0.288675;
-0.288675;
0.288675;
0.288675;
0.000000;
0.000000],1,18,15);

pu_ud = fi(vd_pu(index),1,27,24);
pu_uq = fi(vq_pu(index),1,27,24);
pu_ux = fi(vx_pu(index),1,27,24);
pu_uy = fi(vy_pu(index),1,27,24);
